simulink model "TSR_Scenario_001_cs"  (R2014b)
settings: Solver=ode5  SolverMode=SingleTasking  StartTime=0.0  StopTime=inf  FixedStep=1/100  RelTol=1e-3
PreLoadFcn:
  | mbxruntime.callbacks.PreLoadFcn(bdroot);
  | check_NUTS_defined;
  | 
  | assignin('base',['model_closed_' bdroot],false);
  | 
  | addpath('../includes_TSR/includes_TSR');
  | 
  | switch version('-release')
  | case {'2010a', '2010b', '2011a'}
  | addpath('../includes_TSR/ML2010b');
  | otherwise
  | addpath('../includes_TSR/ML2011b');
  | end
PostLoadFcn:
  | mbxruntime.callbacks.PostLoadFcn(bdroot);
InitFcn:
  | mbxruntime.callbacks.InitFcn(bdroot);
StartFcn:
  | mbxruntime.callbacks.StartFcn(bdroot);
StopFcn:
  | mbxruntime.callbacks.StopFcn(bdroot);
model workspace: external: MAT-File .\TSR_Scenario_001_cs_hws.mat (data not in the file)
undefined symbols (not defined in the file or in its folder): InitImageOutputDir, mbxruntime, OrientationPitch, OrientationRoll, PositionX, PositionY, PositionZ, tabledata, warningInitialVelocity, x0
undefined symbols (not defined in the file): SteeringColumn, SteeringWheel, TSR_Scenario_001_cs_0469e6db089af631, TSR_Scenario_001_cs_0511100212e7bc8e, TSR_Scenario_001_cs_0e7e9ae969427aac, TSR_Scenario_001_cs_1093386e49c2fe1f, TSR_Scenario_001_cs_112063adae8cf595, TSR_Scenario_001_cs_20f00d93cd5331c2, TSR_Scenario_001_cs_23e3512474fbfadc, TSR_Scenario_001_cs_366523e1554c6bf4, TSR_Scenario_001_cs_37bce4982c67337a, TSR_Scenario_001_cs_44e6164a5df50f45, TSR_Scenario_001_cs_4963ce12e7ff3247, TSR_Scenario_001_cs_4b3e01fa729ce73a, TSR_Scenario_001_cs_519c34727ce9f069, TSR_Scenario_001_cs_5b66ab60038399a1, TSR_Scenario_001_cs_5baa165dfa1afdcb, TSR_Scenario_001_cs_5f993ce39fa6372c, TSR_Scenario_001_cs_613fdf28e3ff7437, TSR_Scenario_001_cs_67b1406af835d622, TSR_Scenario_001_cs_6ad990c290286b94, TSR_Scenario_001_cs_6c412b69295984e1, TSR_Scenario_001_cs_6d4c0c06b1585ef3, TSR_Scenario_001_cs_6dd019d071bf1235, TSR_Scenario_001_cs_6e9f5883f1a78533, TSR_Scenario_001_cs_80f7223d9ac35404, TSR_Scenario_001_cs_8562b82d3c89ae57, TSR_Scenario_001_cs_8a3a0181ab0babfe, TSR_Scenario_001_cs_8c997348ce80deaf, TSR_Scenario_001_cs_925bd6a073d9fe25, TSR_Scenario_001_cs_961436216add6114, TSR_Scenario_001_cs_991a7959256b2c84, TSR_Scenario_001_cs_9a95ce2c2e753616, TSR_Scenario_001_cs_a98aa9562e8552a9, TSR_Scenario_001_cs_ab44ae81dbfb58cd, TSR_Scenario_001_cs_Actros_2541_2_Path_pathUniqueID, TSR_Scenario_001_cs_ae74836ade6bff5a, TSR_Scenario_001_cs_Audi_A8_1_Dynamics_Simple_initialPitch, TSR_Scenario_001_cs_Audi_A8_1_Dynamics_Simple_initialRoll, TSR_Scenario_001_cs_Audi_A8_1_Dynamics_Simple_initialX, TSR_Scenario_001_cs_Audi_A8_1_Dynamics_Simple_initialY, TSR_Scenario_001_cs_Audi_A8_1_Dynamics_Simple_initialYaw, TSR_Scenario_001_cs_Audi_A8_1_Dynamics_Simple_initialZ, TSR_Scenario_001_cs_Audi_A8_2_Path_pathUniqueID, TSR_Scenario_001_cs_Audi_A8_2_SpeedProfile_speedProfileUniqueID, TSR_Scenario_001_cs_b2eca4eb2fce349a, TSR_Scenario_001_cs_b7bac209c1f2549f, TSR_Scenario_001_cs_bf3dccb66d3255a4, TSR_Scenario_001_cs_bf4c1a5315e3f716, TSR_Scenario_001_cs_BMW_Z3_1_Path_pathUniqueID, TSR_Scenario_001_cs_BMW_Z3_1_SpeedProfile_speedProfileUniqueID, TSR_Scenario_001_cs_BMW_Z3_2_Path_pathUniqueID, TSR_Scenario_001_cs_BMW_Z3_2_SpeedProfile_speedProfileUniqueID, TSR_Scenario_001_cs_c4c8fc4bdece03a9, TSR_Scenario_001_cs_c964c86aa54ad92e, TSR_Scenario_001_cs_cb64d1ef85329755, TSR_Scenario_001_cs_Citroen_C3_1_Path_pathUniqueID, TSR_Scenario_001_cs_Citroen_C3_2_Path_pathUniqueID, TSR_Scenario_001_cs_Citroen_C3_3_Path_pathUniqueID, TSR_Scenario_001_cs_Citroen_C3_4_Path_pathUniqueID ... (+25)
libraries: simulink x21, PreScanSimulinkLibrary x17, simulink_extras x13
(part 4 of 30)

== system TSR_Scenario_001_cs/Citroen_C3_4 ==
  SELF_Citroen_C3_4 : Inport  Tag=inport/SelfPort  OutDataTypeStr=Bus: PRESCAN_SELFSENSORDATA  PortDimensions=1  SampleTime=1/100  BusOutputAsStruct=on
  ColorRegion_Exterior_color : Constant  Tag=VisuLightConst  Value=[255 240 245]
  Ground_{1..6} (6 alike) : Ground
  JointGroup_WheelDisplacement_V2R : Subsystem  Tag=mux/Wheels  mask(PreScan Velocity to Wheel Angle Block:){TimeStep=1/100, TireRadius=0.29}
      mask prompts: TimeStep "Auto Assigned: Time Step [s]"; TireRadius "Tire Radius [m]"
      settings: DeleteFcn=PreScanBlockDeleteFcn;
      mask Display: disp('Velocity\nto\nWheelAngle')
  Path : S-Function  Tag=Path  LoadFcn=load('PrescanMotionData.mat')  FunctionName=sfun_Path  Parameters=uniqueID, pathUniqueID, timestep  EnableBusSupport=off  mask(Path){uniqueID=2027, pathUniqueID=TSR_Scenario_001_cs_Citroen_C3_4_Path_pathUniqueID, timestep=1/100}
      mask prompts: uniqueID "Object Unique ID"; pathUniqueID "Path Unique ID"; timestep "MATLAB timestep:"
      mask help:
      | The path block outputs the position along a given trajectory.
      |
      | For more information, please click Help.
      mask Help: eval('openHelp(312)')
      mask Display: image(imread('Path.png'))
  SELF_Demux : Subsystem  Tag=demux/SelfPort  mask(PreScan Demux Block:){}
      mask help:
      | The SELF port shows (state) information of the actor itself. The outputs are position in the experiment's axis system and the GPS coordinates, and the object's absolute velocity and compass heading.
      |
      | For more information, please click Help.
      settings: DeleteFcn=PreScanBlockDeleteFcn;
      mask Help: eval('openHelp(462)')
      mask Display:
      | port_label('output',1,'x [m]')
      | port_label('output',2,'y [m]')
      | port_label('output',3,'z [m]','texmode','on')
      | port_label('output',4,'Rotx [deg]','texmode','on')
      | port_label('output',5,'Roty [deg]','texmode','on')
      | port_label('output',6,'Rotz [deg]','texmode','on')
      | port_label('output',7,'GPS lat [deg]','texmode','on')
      | port_label('output',8,'GPS long [deg]','texmode','on')
      | port_label('output',9,'GPS alt [m]','texmode','on')
      | port_label('output',10,'Velocity [m/s]')
      | port_label('output',11,'Heading [deg]')
      | port_label('output',12,'Yaw rate [deg/s]')
  STATE_Citroen_C3_4_rc : RateTransition  Tag=mux_rc/StatePort  OutPortSampleTimeOpt=Inherit
  SpeedProfile : S-Function  Tag=SpeedProfile  LoadFcn=load('PrescanMotionData.mat')  FunctionName=sfun_SpeedProfile  Parameters=speedProfileUniqueID, timestep  EnableBusSupport=off  mask(SpeedProfile){speedProfileUniqueID=TSR_Scenario_001_cs_def3abf47cdc3734, timestep=1/100}
      mask prompts: speedProfileUniqueID "Speed Profile Unique ID"; timestep "MATLAB timestep:"
      mask help:
      | The speed profile block outputs the travelled distance, velocities and acceleration along a given path.
      |
      | For more information, please click Help.
      mask Help: eval('openHelp(312)')
      mask Display: image(imread('SpeedProfile.png'))
  Terminator_{1..11} (11 alike) : Terminator
  VISUColorRegion_Exterior_Mux : Subsystem  Tag=mux/MuxColorRegion  LoadFcn=load PrescanColorData  mask(PreScan User Interface: VisuTextureColor){}
      mask help:
      | The VisuTextureColor block provides a way to adapt the color of a vehicle.
      |
      | For more information, please click Help.
      settings: DeleteFcn=PreScanBlockDeleteFcn;
      mask Help: eval('openHelp(230)')
  WheelDisplacement_Mux : Subsystem  Tag=mux/JointGroup  mask(JointGroup){}
      mask help:
      | The JointGroup allows to control several Joints in one go, as defined for this particular model.
      | For more information, look in the PreScan manual in the section "Model Preparation Tool" -> "Joint Groups"
      |
      | For more information on the Joints simulink interface, press Help.
      mask Help: eval('openHelp(254)')
  STATE_Citroen_C3_4_bus : Outport  Tag=outport/StatePort  OutDataTypeStr=Bus: PRESCAN_STATEACTUATORDATA  PortDimensions=1  SampleTime=1/100
  WheelL0_Citroen_C3_4 : Outport  Tag=outport/JointActuator  Port=2  OutDataTypeStr=Bus: PRESCAN_POSE_DATA  SampleTime=1/100
  WheelL1_Citroen_C3_4 : Outport  Tag=outport/JointActuator  Port=3  OutDataTypeStr=Bus: PRESCAN_POSE_DATA  SampleTime=1/100
  WheelR0_Citroen_C3_4 : Outport  Tag=outport/JointActuator  Port=4  OutDataTypeStr=Bus: PRESCAN_POSE_DATA  SampleTime=1/100
  WheelR1_Citroen_C3_4 : Outport  Tag=outport/JointActuator  Port=5  OutDataTypeStr=Bus: PRESCAN_POSE_DATA  SampleTime=1/100
  VISUColorRegion_Exterior_Citroen_C3_4 : Outport  Tag=outport/ColorRegion  Port=6  OutDataTypeStr=Bus: PRESCAN_COLOR_DATA  PortDimensions=1  SampleTime=1/100
  wires:
  SELF_Demux/10(velocity [m/s]) -> JointGroup_WheelDisplacement_V2R/1(Velocity [m/s])
  STATE_Citroen_C3_4_rc/1 -> STATE_Citroen_C3_4_bus/1
  SpeedProfile/1 -> Path/1
  Path/1 -> STATE_Citroen_C3_4_rc/1
  SELF_Citroen_C3_4/1 -> SELF_Demux/1(SELF)
  WheelDisplacement_Mux/1(WheelL0_Citroen_C3_4) -> WheelL0_Citroen_C3_4/1
  WheelDisplacement_Mux/2(WheelL1_Citroen_C3_4) -> WheelL1_Citroen_C3_4/1
  WheelDisplacement_Mux/3(WheelR0_Citroen_C3_4) -> WheelR0_Citroen_C3_4/1
  WheelDisplacement_Mux/4(WheelR1_Citroen_C3_4) -> WheelR1_Citroen_C3_4/1
  JointGroup_WheelDisplacement_V2R/1(Rotation [rad]) -> WheelDisplacement_Mux/3(Rotation [rad])
  VISUColorRegion_Exterior_Mux/1(ColorRegion) -> VISUColorRegion_Exterior_Citroen_C3_4/1
  ColorRegion_Exterior_color/1 -> VISUColorRegion_Exterior_Mux/1(RGB [-,-,-])
  SELF_Demux/1(x [m]) -> Terminator_1/1
  SELF_Demux/2(y [m]) -> Terminator_2/1
  SELF_Demux/3(z [m]) -> Terminator_3/1
  SELF_Demux/4(rotx [deg]) -> Terminator_4/1
  SELF_Demux/5(roty [deg]) -> Terminator_5/1
  SELF_Demux/6(rotz [deg]) -> Terminator_6/1
  SELF_Demux/7(GPS lat [deg]) -> Terminator_7/1
  SELF_Demux/8(GPS long [deg]) -> Terminator_8/1
  SELF_Demux/9(GPS alt [m]) -> Terminator_9/1
  SELF_Demux/11(heading [deg]) -> Terminator_10/1
  SELF_Demux/12(yaw rate [deg/s]) -> Terminator_11/1
  Ground_1/1 -> WheelDisplacement_Mux/1(Steering Angle Front [rad])
  Ground_2/1 -> WheelDisplacement_Mux/2(Steering Angle Rear [rad])
  Ground_3/1 -> WheelDisplacement_Mux/4(zDisp FL [m])
  Ground_4/1 -> WheelDisplacement_Mux/5(zDisp FR [m])
  Ground_5/1 -> WheelDisplacement_Mux/6(zDisp RL [m])
  Ground_6/1 -> WheelDisplacement_Mux/7(zDisp RR [m])

== system TSR_Scenario_001_cs/ContainerTrailer_DoubleAxle_1 ==
  SELF_ContainerTrailer_DoubleAxle_1 : Inport  Tag=inport/SelfPort  OutDataTypeStr=Bus: PRESCAN_SELFSENSORDATA  PortDimensions=1  SampleTime=1/100  BusOutputAsStruct=on
  ArticulatedActor : S-Function  FunctionName=sfun_ArticulatedActor  Parameters=tractorUniqueID, trailerUniqueID, timestep  EnableBusSupport=off  mask(ArticulatedActor){tractorUniqueID=1580, trailerUniqueID=1582, timestep=1/100}
      mask prompts: tractorUniqueID "Tractor Unique ID"; trailerUniqueID "Trailer Unique ID"; timestep "MATLAB timestep:"
      mask help:
      | The articulated actor block outputs the trailer position.
      |
      | For more information, please click Help.
      mask Help: eval('openHelp(1300)')
      mask Display: image(imread('TrailerKinematics.png'))
  SELF_Demux : Subsystem  Tag=demux/SelfPort  mask(PreScan Demux Block:){}
      mask help:
      | The SELF port shows (state) information of the actor itself. The outputs are position in the experiment's axis system and the GPS coordinates, and the object's absolute velocity and compass heading.
      |
      | For more information, please click Help.
      settings: DeleteFcn=PreScanBlockDeleteFcn;
      mask Help: eval('openHelp(462)')
      mask Display:
      | port_label('output',1,'x [m]')
      | port_label('output',2,'y [m]')
      | port_label('output',3,'z [m]','texmode','on')
      | port_label('output',4,'Rotx [deg]','texmode','on')
      | port_label('output',5,'Roty [deg]','texmode','on')
      | port_label('output',6,'Rotz [deg]','texmode','on')
      | port_label('output',7,'GPS lat [deg]','texmode','on')
      | port_label('output',8,'GPS long [deg]','texmode','on')
      | port_label('output',9,'GPS alt [m]','texmode','on')
      | port_label('output',10,'Velocity [m/s]')
      | port_label('output',11,'Heading [deg]')
      | port_label('output',12,'Yaw rate [deg/s]')
  STATE_ContainerTrailer_DoubleAxle_1_rc : RateTransition  Tag=mux_rc/StatePort  OutPortSampleTimeOpt=Inherit
  Terminator_{1..12} (12 alike) : Terminator
  STATE_ContainerTrailer_DoubleAxle_1_bus : Outport  Tag=outport/StatePort  OutDataTypeStr=Bus: PRESCAN_STATEACTUATORDATA  PortDimensions=1  SampleTime=1/100
  wires:
  STATE_ContainerTrailer_DoubleAxle_1_rc/1 -> STATE_ContainerTrailer_DoubleAxle_1_bus/1
  SELF_ContainerTrailer_DoubleAxle_1/1 -> SELF_Demux/1(SELF)
  ArticulatedActor/1 -> STATE_ContainerTrailer_DoubleAxle_1_rc/1
  [Actros_1860_1_state] -> ArticulatedActor/1
  SELF_Demux/1(x [m]) -> Terminator_1/1
  SELF_Demux/2(y [m]) -> Terminator_2/1
  SELF_Demux/3(z [m]) -> Terminator_3/1
  SELF_Demux/4(rotx [deg]) -> Terminator_4/1
  SELF_Demux/5(roty [deg]) -> Terminator_5/1
  SELF_Demux/6(rotz [deg]) -> Terminator_6/1
  SELF_Demux/7(GPS lat [deg]) -> Terminator_7/1
  SELF_Demux/8(GPS long [deg]) -> Terminator_8/1
  SELF_Demux/9(GPS alt [m]) -> Terminator_9/1
  SELF_Demux/10(velocity [m/s]) -> Terminator_10/1
  SELF_Demux/11(heading [deg]) -> Terminator_11/1
  SELF_Demux/12(yaw rate [deg/s]) -> Terminator_12/1

== system TSR_Scenario_001_cs/ContainerTrailer_DoubleAxle_2 ==
  SELF_ContainerTrailer_DoubleAxle_2 : Inport  Tag=inport/SelfPort  OutDataTypeStr=Bus: PRESCAN_SELFSENSORDATA  PortDimensions=1  SampleTime=1/100  BusOutputAsStruct=on
  ArticulatedActor : S-Function  FunctionName=sfun_ArticulatedActor  Parameters=tractorUniqueID, trailerUniqueID, timestep  EnableBusSupport=off  mask(ArticulatedActor){tractorUniqueID=1584, trailerUniqueID=1586, timestep=1/100}
      mask prompts: tractorUniqueID "Tractor Unique ID"; trailerUniqueID "Trailer Unique ID"; timestep "MATLAB timestep:"
      mask help:
      | The articulated actor block outputs the trailer position.
      |
      | For more information, please click Help.
      mask Help: eval('openHelp(1300)')
      mask Display: image(imread('TrailerKinematics.png'))
  SELF_Demux : Subsystem  Tag=demux/SelfPort  mask(PreScan Demux Block:){}
      mask help:
      | The SELF port shows (state) information of the actor itself. The outputs are position in the experiment's axis system and the GPS coordinates, and the object's absolute velocity and compass heading.
      |
      | For more information, please click Help.
      settings: DeleteFcn=PreScanBlockDeleteFcn;
      mask Help: eval('openHelp(462)')
      mask Display:
      | port_label('output',1,'x [m]')
      | port_label('output',2,'y [m]')
      | port_label('output',3,'z [m]','texmode','on')
      | port_label('output',4,'Rotx [deg]','texmode','on')
      | port_label('output',5,'Roty [deg]','texmode','on')
      | port_label('output',6,'Rotz [deg]','texmode','on')
      | port_label('output',7,'GPS lat [deg]','texmode','on')
      | port_label('output',8,'GPS long [deg]','texmode','on')
      | port_label('output',9,'GPS alt [m]','texmode','on')
      | port_label('output',10,'Velocity [m/s]')
      | port_label('output',11,'Heading [deg]')
      | port_label('output',12,'Yaw rate [deg/s]')
  STATE_ContainerTrailer_DoubleAxle_2_rc : RateTransition  Tag=mux_rc/StatePort  OutPortSampleTimeOpt=Inherit
  Terminator_{1..12} (12 alike) : Terminator
  STATE_ContainerTrailer_DoubleAxle_2_bus : Outport  Tag=outport/StatePort  OutDataTypeStr=Bus: PRESCAN_STATEACTUATORDATA  PortDimensions=1  SampleTime=1/100
  wires:
  STATE_ContainerTrailer_DoubleAxle_2_rc/1 -> STATE_ContainerTrailer_DoubleAxle_2_bus/1
  SELF_ContainerTrailer_DoubleAxle_2/1 -> SELF_Demux/1(SELF)
  ArticulatedActor/1 -> STATE_ContainerTrailer_DoubleAxle_2_rc/1
  [Actros_1860_2_state] -> ArticulatedActor/1
  SELF_Demux/1(x [m]) -> Terminator_1/1
  SELF_Demux/2(y [m]) -> Terminator_2/1
  SELF_Demux/3(z [m]) -> Terminator_3/1
  SELF_Demux/4(rotx [deg]) -> Terminator_4/1
  SELF_Demux/5(roty [deg]) -> Terminator_5/1
  SELF_Demux/6(rotz [deg]) -> Terminator_6/1
  SELF_Demux/7(GPS lat [deg]) -> Terminator_7/1
  SELF_Demux/8(GPS long [deg]) -> Terminator_8/1
  SELF_Demux/9(GPS alt [m]) -> Terminator_9/1
  SELF_Demux/10(velocity [m/s]) -> Terminator_10/1
  SELF_Demux/11(heading [deg]) -> Terminator_11/1
  SELF_Demux/12(yaw rate [deg/s]) -> Terminator_12/1

== system TSR_Scenario_001_cs/Controller ==
  Terminator : Terminator
  sfun_Controller : S-Function  FunctionName=sfun_Controller  Parameters=SParameter1, SParameter2, SParameter3, SParameter4, SParameter5, SParameter6, SParameter7, SParameter8, SParameter9, SParameter10, SampleTime  EnableBusSupport=off  mask(Legacy Function){SFunctionSpec=void prescan_outputFcn(void** work1, PRESCAN_CONTROLLERDATA y1[1]), SParameter1=uint8([ExperimentFile 0]), SParameter2=uint8([ModelDepo 0]), SParameter3=uint8([ControllerOptions 0]), SParameter4=RTmode, SParameter5=PreScanExecutionMode, SParameter6=ControlMode, SParameter7=ControllerCount, SParameter8=ControllerIndex, SParameter9=uint8([SimulationMode 0]), SParameter10=uint8([TargetName 0]), SampleTime=TimeStep, ShowSpec=on}
      mask prompts: SParameter1 "P1:"; SParameter2 "P2:"; SParameter3 "P3:"; SParameter4 "P4:"; SParameter5 "P5:"; SParameter6 "P6:"; SParameter7 "P7:"; SParameter8 "P8:"; SParameter9 "P9:"; SParameter10 "P10:"; SampleTime "Sample time (-1 for inherited):"; ShowSpec "Display function specification"
      mask help:
      | This block allows you to call the legacy functions specified by the following Legacy Code Tool definition:
      | def.SFunctionName = 'sfun_Controller';
      | def.OutputFcnSpec = 'void prescan_outputFcn(void** work1, PRESCAN_CONTROLLERDATA y1[1])';
      | def.StartFcnSpec = 'void prescan_startFcn(void ** work1, uint8 p1[], uint8 p2[], uint8 p3[], double p4, double p5, double p6, double p7, double p8, uint8 p9[], uint8 p10[])';
      | def.TerminateFcnSpec = 'void prescan_terminateFcn(void** work1)';
      | def.HeaderFiles = {'prescan_controller_data.h', 'prescan_SFunLibrary.h', 'prescan_CreateLogHandler.h', 'prescan_CreateErrorHandler.h', 'prescan_modify.h', 'ModuleDLL.h'};
      | def.SourceFiles = {'prescan_MexLogHandler.c', 'prescan_SimStructErrorHandler.c', 'prescan_LogHandler.c', 'prescan_ErrorHandler.c', 'prescan_Modify.c'};
      | def.HostLibFiles = {'sensorinterfaced.lib'};
      | def.TargetLibFiles = {'sensorinterfaced.so'};
      | def.IncPaths = {'.', 'C:\projects\prescan\rt_vislibrary\vis\..\pimp\include\sensors\InterfaceRTW'};
      | def.SrcPaths = {'C:\projects\prescan\rt_vislibrary\vis\..\pimp\include\sensors\InterfaceRTW', 'C:\projects\prescan\rt_vislibrary\vis\..\pimp\include\sensors\InterfaceRTW\ccurrt'};
      | def.LibPaths = {'C:\\projects\\prescan\\vislibrary_build\lib'};
      | def.SampleTime = 'parameterized';
      mask Help: <p>This block was generated automatically by the Legacy Code Tool. For detailed help on this tool, call<a href="matlab:legacy_code('help')"> legacy_code('help')</a>.</p>
      mask Callback ShowSpec:
      | if strcmp(get_param(gcbh, 'ShowSpec'), 'on')
      |   set_param(gcbh, 'MaskDisplay', sprintf('fprintf(''%s'');', get_param(gcbh, 'SFunctionSpec')));
      | else
      |   set_param(gcbh, 'MaskDisplay', sprintf('fprintf(''%s'');', get_param(gcbh, 'FunctionName')));
      | end
      mask Display: fprintf('void prescan_outputFcn(void** work1, PRESCAN_CONTROLLERDATA y1[1])');
  wires:
  sfun_Controller/1 -> Terminator/1

== system TSR_Scenario_001_cs/Fiat_Bravo_1 ==
  SELF_Fiat_Bravo_1 : Inport  Tag=inport/SelfPort  OutDataTypeStr=Bus: PRESCAN_SELFSENSORDATA  PortDimensions=1  SampleTime=1/100  BusOutputAsStruct=on
  ColorRegion_Exterior_color : Constant  Tag=VisuLightConst  Value=[0 191 255]
  Ground_{1..6} (6 alike) : Ground
  JointGroup_WheelDisplacement_V2R : Subsystem  Tag=mux/Wheels  mask(PreScan Velocity to Wheel Angle Block:){TimeStep=1/100, TireRadius=0.29}
      mask prompts: TimeStep "Auto Assigned: Time Step [s]"; TireRadius "Tire Radius [m]"
      settings: DeleteFcn=PreScanBlockDeleteFcn;
      mask Display: disp('Velocity\nto\nWheelAngle')
  Path : S-Function  Tag=Path  LoadFcn=load('PrescanMotionData.mat')  FunctionName=sfun_Path  Parameters=uniqueID, pathUniqueID, timestep  EnableBusSupport=off  mask(Path){uniqueID=1964, pathUniqueID=TSR_Scenario_001_cs_Fiat_Bravo_1_Path_pathUniqueID, timestep=1/100}
      mask prompts: uniqueID "Object Unique ID"; pathUniqueID "Path Unique ID"; timestep "MATLAB timestep:"
      mask help:
      | The path block outputs the position along a given trajectory.
      |
      | For more information, please click Help.
      mask Help: eval('openHelp(312)')
      mask Display: image(imread('Path.png'))
  SELF_Demux : Subsystem  Tag=demux/SelfPort  mask(PreScan Demux Block:){}
      mask help:
      | The SELF port shows (state) information of the actor itself. The outputs are position in the experiment's axis system and the GPS coordinates, and the object's absolute velocity and compass heading.
      |
      | For more information, please click Help.
      settings: DeleteFcn=PreScanBlockDeleteFcn;
      mask Help: eval('openHelp(462)')
      mask Display:
      | port_label('output',1,'x [m]')
      | port_label('output',2,'y [m]')
      | port_label('output',3,'z [m]','texmode','on')
      | port_label('output',4,'Rotx [deg]','texmode','on')
      | port_label('output',5,'Roty [deg]','texmode','on')
      | port_label('output',6,'Rotz [deg]','texmode','on')
      | port_label('output',7,'GPS lat [deg]','texmode','on')
      | port_label('output',8,'GPS long [deg]','texmode','on')
      | port_label('output',9,'GPS alt [m]','texmode','on')
      | port_label('output',10,'Velocity [m/s]')
      | port_label('output',11,'Heading [deg]')
      | port_label('output',12,'Yaw rate [deg/s]')
  STATE_Fiat_Bravo_1_rc : RateTransition  Tag=mux_rc/StatePort  OutPortSampleTimeOpt=Inherit
  SpeedProfile : S-Function  Tag=SpeedProfile  LoadFcn=load('PrescanMotionData.mat')  FunctionName=sfun_SpeedProfile  Parameters=speedProfileUniqueID, timestep  EnableBusSupport=off  mask(SpeedProfile){speedProfileUniqueID=TSR_Scenario_001_cs_fb6cb42c10e88917, timestep=1/100}
      mask prompts: speedProfileUniqueID "Speed Profile Unique ID"; timestep "MATLAB timestep:"
      mask help:
      | The speed profile block outputs the travelled distance, velocities and acceleration along a given path.
      |
      | For more information, please click Help.
      mask Help: eval('openHelp(312)')
      mask Display: image(imread('SpeedProfile.png'))
  Terminator_{1..11} (11 alike) : Terminator
  VISUColorRegion_Exterior_Mux : Subsystem  Tag=mux/MuxColorRegion  LoadFcn=load PrescanColorData  mask(PreScan User Interface: VisuTextureColor){}
      mask help:
      | The VisuTextureColor block provides a way to adapt the color of a vehicle.
      |
      | For more information, please click Help.
      settings: DeleteFcn=PreScanBlockDeleteFcn;
      mask Help: eval('openHelp(230)')
  WheelDisplacement_Mux : Subsystem  Tag=mux/JointGroup  mask(JointGroup){}
      mask help:
      | The JointGroup allows to control several Joints in one go, as defined for this particular model.
      | For more information, look in the PreScan manual in the section "Model Preparation Tool" -> "Joint Groups"
      |
      | For more information on the Joints simulink interface, press Help.
      mask Help: eval('openHelp(254)')
  STATE_Fiat_Bravo_1_bus : Outport  Tag=outport/StatePort  OutDataTypeStr=Bus: PRESCAN_STATEACTUATORDATA  PortDimensions=1  SampleTime=1/100
  WheelL0_Fiat_Bravo_1 : Outport  Tag=outport/JointActuator  Port=2  OutDataTypeStr=Bus: PRESCAN_POSE_DATA  SampleTime=1/100
  WheelL1_Fiat_Bravo_1 : Outport  Tag=outport/JointActuator  Port=3  OutDataTypeStr=Bus: PRESCAN_POSE_DATA  SampleTime=1/100
  WheelR0_Fiat_Bravo_1 : Outport  Tag=outport/JointActuator  Port=4  OutDataTypeStr=Bus: PRESCAN_POSE_DATA  SampleTime=1/100
  WheelR1_Fiat_Bravo_1 : Outport  Tag=outport/JointActuator  Port=5  OutDataTypeStr=Bus: PRESCAN_POSE_DATA  SampleTime=1/100
  VISUColorRegion_Exterior_Fiat_Bravo_1 : Outport  Tag=outport/ColorRegion  Port=6  OutDataTypeStr=Bus: PRESCAN_COLOR_DATA  PortDimensions=1  SampleTime=1/100
  wires:
  SELF_Demux/10(velocity [m/s]) -> JointGroup_WheelDisplacement_V2R/1(Velocity [m/s])
  STATE_Fiat_Bravo_1_rc/1 -> STATE_Fiat_Bravo_1_bus/1
  SpeedProfile/1 -> Path/1
  Path/1 -> STATE_Fiat_Bravo_1_rc/1
  SELF_Fiat_Bravo_1/1 -> SELF_Demux/1(SELF)
  WheelDisplacement_Mux/1(WheelL0_Fiat_Bravo_1) -> WheelL0_Fiat_Bravo_1/1
  WheelDisplacement_Mux/2(WheelL1_Fiat_Bravo_1) -> WheelL1_Fiat_Bravo_1/1
  WheelDisplacement_Mux/3(WheelR0_Fiat_Bravo_1) -> WheelR0_Fiat_Bravo_1/1
  WheelDisplacement_Mux/4(WheelR1_Fiat_Bravo_1) -> WheelR1_Fiat_Bravo_1/1
  JointGroup_WheelDisplacement_V2R/1(Rotation [rad]) -> WheelDisplacement_Mux/3(Rotation [rad])
  VISUColorRegion_Exterior_Mux/1(ColorRegion) -> VISUColorRegion_Exterior_Fiat_Bravo_1/1
  ColorRegion_Exterior_color/1 -> VISUColorRegion_Exterior_Mux/1(RGB [-,-,-])
  SELF_Demux/1(x [m]) -> Terminator_1/1
  SELF_Demux/2(y [m]) -> Terminator_2/1
  SELF_Demux/3(z [m]) -> Terminator_3/1
  SELF_Demux/4(rotx [deg]) -> Terminator_4/1
  SELF_Demux/5(roty [deg]) -> Terminator_5/1
  SELF_Demux/6(rotz [deg]) -> Terminator_6/1
  SELF_Demux/7(GPS lat [deg]) -> Terminator_7/1
  SELF_Demux/8(GPS long [deg]) -> Terminator_8/1
  SELF_Demux/9(GPS alt [m]) -> Terminator_9/1
  SELF_Demux/11(heading [deg]) -> Terminator_10/1
  SELF_Demux/12(yaw rate [deg/s]) -> Terminator_11/1
  Ground_1/1 -> WheelDisplacement_Mux/1(Steering Angle Front [rad])
  Ground_2/1 -> WheelDisplacement_Mux/2(Steering Angle Rear [rad])
  Ground_3/1 -> WheelDisplacement_Mux/4(zDisp FL [m])
  Ground_4/1 -> WheelDisplacement_Mux/5(zDisp FR [m])
  Ground_5/1 -> WheelDisplacement_Mux/6(zDisp RL [m])
  Ground_6/1 -> WheelDisplacement_Mux/7(zDisp RR [m])

== system TSR_Scenario_001_cs/Fiat_Bravo_2 ==
  SELF_Fiat_Bravo_2 : Inport  Tag=inport/SelfPort  OutDataTypeStr=Bus: PRESCAN_SELFSENSORDATA  PortDimensions=1  SampleTime=1/100  BusOutputAsStruct=on
  Ground_{1..6} (6 alike) : Ground
  JointGroup_WheelDisplacement_V2R : Subsystem  Tag=mux/Wheels  mask(PreScan Velocity to Wheel Angle Block:){TimeStep=1/100, TireRadius=0.29}
      mask prompts: TimeStep "Auto Assigned: Time Step [s]"; TireRadius "Tire Radius [m]"
      settings: DeleteFcn=PreScanBlockDeleteFcn;
      mask Display: disp('Velocity\nto\nWheelAngle')
  Path : S-Function  Tag=Path  LoadFcn=load('PrescanMotionData.mat')  FunctionName=sfun_Path  Parameters=uniqueID, pathUniqueID, timestep  EnableBusSupport=off  mask(Path){uniqueID=2021, pathUniqueID=TSR_Scenario_001_cs_Fiat_Bravo_2_Path_pathUniqueID, timestep=1/100}
      mask prompts: uniqueID "Object Unique ID"; pathUniqueID "Path Unique ID"; timestep "MATLAB timestep:"
      mask help:
      | The path block outputs the position along a given trajectory.
      |
      | For more information, please click Help.
      mask Help: eval('openHelp(312)')
      mask Display: image(imread('Path.png'))
  SELF_Demux : Subsystem  Tag=demux/SelfPort  mask(PreScan Demux Block:){}
      mask help:
      | The SELF port shows (state) information of the actor itself. The outputs are position in the experiment's axis system and the GPS coordinates, and the object's absolute velocity and compass heading.
      |
      | For more information, please click Help.
      settings: DeleteFcn=PreScanBlockDeleteFcn;
      mask Help: eval('openHelp(462)')
      mask Display:
      | port_label('output',1,'x [m]')
      | port_label('output',2,'y [m]')
      | port_label('output',3,'z [m]','texmode','on')
      | port_label('output',4,'Rotx [deg]','texmode','on')
      | port_label('output',5,'Roty [deg]','texmode','on')
      | port_label('output',6,'Rotz [deg]','texmode','on')
      | port_label('output',7,'GPS lat [deg]','texmode','on')
      | port_label('output',8,'GPS long [deg]','texmode','on')
      | port_label('output',9,'GPS alt [m]','texmode','on')
      | port_label('output',10,'Velocity [m/s]')
      | port_label('output',11,'Heading [deg]')
      | port_label('output',12,'Yaw rate [deg/s]')
  STATE_Fiat_Bravo_2_rc : RateTransition  Tag=mux_rc/StatePort  OutPortSampleTimeOpt=Inherit
  SpeedProfile : S-Function  Tag=SpeedProfile  LoadFcn=load('PrescanMotionData.mat')  FunctionName=sfun_SpeedProfile  Parameters=speedProfileUniqueID, timestep  EnableBusSupport=off  mask(SpeedProfile){speedProfileUniqueID=TSR_Scenario_001_cs_fd67c8a405d181e0, timestep=1/100}
      mask prompts: speedProfileUniqueID "Speed Profile Unique ID"; timestep "MATLAB timestep:"
      mask help:
      | The speed profile block outputs the travelled distance, velocities and acceleration along a given path.
      |
      | For more information, please click Help.
      mask Help: eval('openHelp(312)')
      mask Display: image(imread('SpeedProfile.png'))
  Terminator_{1..11} (11 alike) : Terminator
  WheelDisplacement_Mux : Subsystem  Tag=mux/JointGroup  mask(JointGroup){}
      mask help:
      | The JointGroup allows to control several Joints in one go, as defined for this particular model.
      | For more information, look in the PreScan manual in the section "Model Preparation Tool" -> "Joint Groups"
      |
      | For more information on the Joints simulink interface, press Help.
      mask Help: eval('openHelp(254)')
  STATE_Fiat_Bravo_2_bus : Outport  Tag=outport/StatePort  OutDataTypeStr=Bus: PRESCAN_STATEACTUATORDATA  PortDimensions=1  SampleTime=1/100
  WheelL0_Fiat_Bravo_2 : Outport  Tag=outport/JointActuator  Port=2  OutDataTypeStr=Bus: PRESCAN_POSE_DATA  SampleTime=1/100
  WheelL1_Fiat_Bravo_2 : Outport  Tag=outport/JointActuator  Port=3  OutDataTypeStr=Bus: PRESCAN_POSE_DATA  SampleTime=1/100
  WheelR0_Fiat_Bravo_2 : Outport  Tag=outport/JointActuator  Port=4  OutDataTypeStr=Bus: PRESCAN_POSE_DATA  SampleTime=1/100
  WheelR1_Fiat_Bravo_2 : Outport  Tag=outport/JointActuator  Port=5  OutDataTypeStr=Bus: PRESCAN_POSE_DATA  SampleTime=1/100
  wires:
  SELF_Demux/10(velocity [m/s]) -> JointGroup_WheelDisplacement_V2R/1(Velocity [m/s])
  STATE_Fiat_Bravo_2_rc/1 -> STATE_Fiat_Bravo_2_bus/1
  SpeedProfile/1 -> Path/1
  Path/1 -> STATE_Fiat_Bravo_2_rc/1
  SELF_Fiat_Bravo_2/1 -> SELF_Demux/1(SELF)
  WheelDisplacement_Mux/1(WheelL0_Fiat_Bravo_2) -> WheelL0_Fiat_Bravo_2/1
  WheelDisplacement_Mux/2(WheelL1_Fiat_Bravo_2) -> WheelL1_Fiat_Bravo_2/1
  WheelDisplacement_Mux/3(WheelR0_Fiat_Bravo_2) -> WheelR0_Fiat_Bravo_2/1
  WheelDisplacement_Mux/4(WheelR1_Fiat_Bravo_2) -> WheelR1_Fiat_Bravo_2/1
  JointGroup_WheelDisplacement_V2R/1(Rotation [rad]) -> WheelDisplacement_Mux/3(Rotation [rad])
  SELF_Demux/1(x [m]) -> Terminator_1/1
  SELF_Demux/2(y [m]) -> Terminator_2/1
  SELF_Demux/3(z [m]) -> Terminator_3/1
  SELF_Demux/4(rotx [deg]) -> Terminator_4/1
  SELF_Demux/5(roty [deg]) -> Terminator_5/1
  SELF_Demux/6(rotz [deg]) -> Terminator_6/1
  SELF_Demux/7(GPS lat [deg]) -> Terminator_7/1
  SELF_Demux/8(GPS long [deg]) -> Terminator_8/1
  SELF_Demux/9(GPS alt [m]) -> Terminator_9/1
  SELF_Demux/11(heading [deg]) -> Terminator_10/1
  SELF_Demux/12(yaw rate [deg/s]) -> Terminator_11/1
  Ground_1/1 -> WheelDisplacement_Mux/1(Steering Angle Front [rad])
  Ground_2/1 -> WheelDisplacement_Mux/2(Steering Angle Rear [rad])
  Ground_3/1 -> WheelDisplacement_Mux/4(zDisp FL [m])
  Ground_4/1 -> WheelDisplacement_Mux/5(zDisp FR [m])
  Ground_5/1 -> WheelDisplacement_Mux/6(zDisp RL [m])
  Ground_6/1 -> WheelDisplacement_Mux/7(zDisp RR [m])

== system TSR_Scenario_001_cs/Ford_Fiesta_1 ==
  SELF_Ford_Fiesta_1 : Inport  Tag=inport/SelfPort  OutDataTypeStr=Bus: PRESCAN_SELFSENSORDATA  PortDimensions=1  SampleTime=1/100  BusOutputAsStruct=on
  ColorRegion_Exterior_color : Constant  Tag=VisuLightConst  Value=[210 105 30]
  Ground_{1..6} (6 alike) : Ground
  JointGroup_WheelDisplacement_V2R : Subsystem  Tag=mux/Wheels  mask(PreScan Velocity to Wheel Angle Block:){TimeStep=1/100, TireRadius=0.29}
      mask prompts: TimeStep "Auto Assigned: Time Step [s]"; TireRadius "Tire Radius [m]"
      settings: DeleteFcn=PreScanBlockDeleteFcn;
      mask Display: disp('Velocity\nto\nWheelAngle')
  Path : S-Function  Tag=Path  LoadFcn=load('PrescanMotionData.mat')  FunctionName=sfun_Path  Parameters=uniqueID, pathUniqueID, timestep  EnableBusSupport=off  mask(Path){uniqueID=1934, pathUniqueID=TSR_Scenario_001_cs_Ford_Fiesta_1_Path_pathUniqueID, timestep=1/100}
      mask prompts: uniqueID "Object Unique ID"; pathUniqueID "Path Unique ID"; timestep "MATLAB timestep:"
      mask help:
      | The path block outputs the position along a given trajectory.
      |
      | For more information, please click Help.
      mask Help: eval('openHelp(312)')
      mask Display: image(imread('Path.png'))
  SELF_Demux : Subsystem  Tag=demux/SelfPort  mask(PreScan Demux Block:){}
      mask help:
      | The SELF port shows (state) information of the actor itself. The outputs are position in the experiment's axis system and the GPS coordinates, and the object's absolute velocity and compass heading.
      |
      | For more information, please click Help.
      settings: DeleteFcn=PreScanBlockDeleteFcn;
      mask Help: eval('openHelp(462)')
      mask Display:
      | port_label('output',1,'x [m]')
      | port_label('output',2,'y [m]')
      | port_label('output',3,'z [m]','texmode','on')
      | port_label('output',4,'Rotx [deg]','texmode','on')
      | port_label('output',5,'Roty [deg]','texmode','on')
      | port_label('output',6,'Rotz [deg]','texmode','on')
      | port_label('output',7,'GPS lat [deg]','texmode','on')
      | port_label('output',8,'GPS long [deg]','texmode','on')
      | port_label('output',9,'GPS alt [m]','texmode','on')
      | port_label('output',10,'Velocity [m/s]')
      | port_label('output',11,'Heading [deg]')
      | port_label('output',12,'Yaw rate [deg/s]')
  STATE_Ford_Fiesta_1_rc : RateTransition  Tag=mux_rc/StatePort  OutPortSampleTimeOpt=Inherit
  SpeedProfile : S-Function  Tag=SpeedProfile  LoadFcn=load('PrescanMotionData.mat')  FunctionName=sfun_SpeedProfile  Parameters=speedProfileUniqueID, timestep  EnableBusSupport=off  mask(SpeedProfile){speedProfileUniqueID=TSR_Scenario_001_cs_c964c86aa54ad92e, timestep=1/100}
      mask prompts: speedProfileUniqueID "Speed Profile Unique ID"; timestep "MATLAB timestep:"
      mask help:
      | The speed profile block outputs the travelled distance, velocities and acceleration along a given path.
      |
      | For more information, please click Help.
      mask Help: eval('openHelp(312)')
      mask Display: image(imread('SpeedProfile.png'))
  Terminator_{1..11} (11 alike) : Terminator
  VISUColorRegion_Exterior_Mux : Subsystem  Tag=mux/MuxColorRegion  LoadFcn=load PrescanColorData  mask(PreScan User Interface: VisuTextureColor){}
      mask help:
      | The VisuTextureColor block provides a way to adapt the color of a vehicle.
      |
      | For more information, please click Help.
      settings: DeleteFcn=PreScanBlockDeleteFcn;
      mask Help: eval('openHelp(230)')
  WheelDisplacement_Mux : Subsystem  Tag=mux/JointGroup  mask(JointGroup){}
      mask help:
      | The JointGroup allows to control several Joints in one go, as defined for this particular model.
      | For more information, look in the PreScan manual in the section "Model Preparation Tool" -> "Joint Groups"
      |
      | For more information on the Joints simulink interface, press Help.
      mask Help: eval('openHelp(254)')
  STATE_Ford_Fiesta_1_bus : Outport  Tag=outport/StatePort  OutDataTypeStr=Bus: PRESCAN_STATEACTUATORDATA  PortDimensions=1  SampleTime=1/100
  WheelL0_Ford_Fiesta_1 : Outport  Tag=outport/JointActuator  Port=2  OutDataTypeStr=Bus: PRESCAN_POSE_DATA  SampleTime=1/100
  WheelL1_Ford_Fiesta_1 : Outport  Tag=outport/JointActuator  Port=3  OutDataTypeStr=Bus: PRESCAN_POSE_DATA  SampleTime=1/100
  WheelR0_Ford_Fiesta_1 : Outport  Tag=outport/JointActuator  Port=4  OutDataTypeStr=Bus: PRESCAN_POSE_DATA  SampleTime=1/100
  WheelR1_Ford_Fiesta_1 : Outport  Tag=outport/JointActuator  Port=5  OutDataTypeStr=Bus: PRESCAN_POSE_DATA  SampleTime=1/100
  VISUColorRegion_Exterior_Ford_Fiesta_1 : Outport  Tag=outport/ColorRegion  Port=6  OutDataTypeStr=Bus: PRESCAN_COLOR_DATA  PortDimensions=1  SampleTime=1/100
  wires:
  SELF_Demux/10(velocity [m/s]) -> JointGroup_WheelDisplacement_V2R/1(Velocity [m/s])
  STATE_Ford_Fiesta_1_rc/1 -> STATE_Ford_Fiesta_1_bus/1
  SpeedProfile/1 -> Path/1
  Path/1 -> STATE_Ford_Fiesta_1_rc/1
  SELF_Ford_Fiesta_1/1 -> SELF_Demux/1(SELF)
  WheelDisplacement_Mux/1(WheelL0_Ford_Fiesta_1) -> WheelL0_Ford_Fiesta_1/1
  WheelDisplacement_Mux/2(WheelL1_Ford_Fiesta_1) -> WheelL1_Ford_Fiesta_1/1
  WheelDisplacement_Mux/3(WheelR0_Ford_Fiesta_1) -> WheelR0_Ford_Fiesta_1/1
  WheelDisplacement_Mux/4(WheelR1_Ford_Fiesta_1) -> WheelR1_Ford_Fiesta_1/1
  JointGroup_WheelDisplacement_V2R/1(Rotation [rad]) -> WheelDisplacement_Mux/3(Rotation [rad])
  VISUColorRegion_Exterior_Mux/1(ColorRegion) -> VISUColorRegion_Exterior_Ford_Fiesta_1/1
  ColorRegion_Exterior_color/1 -> VISUColorRegion_Exterior_Mux/1(RGB [-,-,-])
  SELF_Demux/1(x [m]) -> Terminator_1/1
  SELF_Demux/2(y [m]) -> Terminator_2/1
  SELF_Demux/3(z [m]) -> Terminator_3/1
  SELF_Demux/4(rotx [deg]) -> Terminator_4/1
  SELF_Demux/5(roty [deg]) -> Terminator_5/1
  SELF_Demux/6(rotz [deg]) -> Terminator_6/1
  SELF_Demux/7(GPS lat [deg]) -> Terminator_7/1
  SELF_Demux/8(GPS long [deg]) -> Terminator_8/1
  SELF_Demux/9(GPS alt [m]) -> Terminator_9/1
  SELF_Demux/11(heading [deg]) -> Terminator_10/1
  SELF_Demux/12(yaw rate [deg/s]) -> Terminator_11/1
  Ground_1/1 -> WheelDisplacement_Mux/1(Steering Angle Front [rad])
  Ground_2/1 -> WheelDisplacement_Mux/2(Steering Angle Rear [rad])
  Ground_3/1 -> WheelDisplacement_Mux/4(zDisp FL [m])
  Ground_4/1 -> WheelDisplacement_Mux/5(zDisp FR [m])
  Ground_5/1 -> WheelDisplacement_Mux/6(zDisp RL [m])
  Ground_6/1 -> WheelDisplacement_Mux/7(zDisp RR [m])

== system TSR_Scenario_001_cs/HighwayOverhang_1 ==
  note: Resources
      |
      | 3: InformationSign\MatrixSign_Empty.png: MatrixSign Empty
      | 4: InformationSign\MatrixSign_End.png: MatrixSign End
      | 5: InformationSign\MatrixSign_GreenArrow.png: MatrixSign GreenArrow
      | 6: InformationSign\MatrixSign_RedCross.png: MatrixSign RedCross
      | 7: InformationSign\MatrixSign_Speed_50.png: MatrixSign Speed 50
      | 8: InformationSign\MatrixSign_Speed_70.png: MatrixSign Speed 70
      | 9: InformationSign\MatrixSign_Speed_90.png: MatrixSign Speed 90
      | 10: InformationSign\MatrixSign_Speed_120.png: MatrixSign Speed 120
      | 11: InformationSign\MatrixSign_Speed_130.png: MatrixSign Speed 130
      | 12: InformationSign\information.png: information
      | 13: InformationSign\Empty.jpg: Empty
  Ground_{1..8} (8 alike) : Ground
  VISUMatrixSignLights_Mux : Subsystem  Tag=mux/VisuMatrixSignLights  mask(PreScan User Interface: VisuMatrixSignLights){}
      mask help:
      | The VisuMatrixSignLights block provides a way to switch the lights on the matrix sign board on or off
      |
      | For more information, please click Help.
      mask Help: eval('openHelp(732)')
  VISUMatrixSign_Mux : Subsystem  Tag=mux/MatrixSign_v2  mask(PreScan User Interface: VisuMatrixSign){}
      mask help:
      | The VisuMatrixSign block provides a way to adapt the texture of the plates connected to an overhang, based on Resource IDs of the texture files.
      |
      | For more information, please click Help.
      settings: DeleteFcn=PreScanBlockDeleteFcn;
      mask Help: eval('openHelp(733)')
  VISUMatrixSign_HighwayOverhang_1 : Outport  Tag=outport/VisuMatrixSign  SampleTime=1/100
  VISUMatrixSignLights_HighwayOverhang_1 : Outport  Tag=outport/VisuMatrixSignLights  Port=2  SampleTime=1/100
  wires:
  VISUMatrixSign_Mux/1(MatrixSigns) -> VISUMatrixSign_HighwayOverhang_1/1
  VISUMatrixSignLights_Mux/1(VISUMatrixSignLights_HighwayOverhang_1) -> VISUMatrixSignLights_HighwayOverhang_1/1
  Ground_1/1 -> VISUMatrixSignLights_Mux/1(MatrixSign_1)
  Ground_2/1 -> VISUMatrixSignLights_Mux/2(MatrixSign_2)
  Ground_3/1 -> VISUMatrixSignLights_Mux/3(MatrixSign_3)
  Ground_4/1 -> VISUMatrixSignLights_Mux/4(MatrixSign_4)
  Ground_5/1 -> VISUMatrixSign_Mux/1(MatrixSign_1)
  Ground_6/1 -> VISUMatrixSign_Mux/2(MatrixSign_2)
  Ground_7/1 -> VISUMatrixSign_Mux/3(MatrixSign_3)
  Ground_8/1 -> VISUMatrixSign_Mux/4(MatrixSign_4)

== system TSR_Scenario_001_cs/HighwayOverhang_2 ==
  note: Resources
      |
      | 3: InformationSign\MatrixSign_Empty.png: MatrixSign Empty
      | 4: InformationSign\MatrixSign_End.png: MatrixSign End
      | 5: InformationSign\MatrixSign_GreenArrow.png: MatrixSign GreenArrow
      | 6: InformationSign\MatrixSign_RedCross.png: MatrixSign RedCross
      | 7: InformationSign\MatrixSign_Speed_50.png: MatrixSign Speed 50
      | 8: InformationSign\MatrixSign_Speed_70.png: MatrixSign Speed 70
      | 9: InformationSign\MatrixSign_Speed_90.png: MatrixSign Speed 90
      | 10: InformationSign\MatrixSign_Speed_120.png: MatrixSign Speed 120
      | 11: InformationSign\MatrixSign_Speed_130.png: MatrixSign Speed 130
      | 12: InformationSign\information.png: information
      | 13: InformationSign\Empty.jpg: Empty
  Ground_{1..8} (8 alike) : Ground
  VISUMatrixSignLights_Mux : Subsystem  Tag=mux/VisuMatrixSignLights  mask(PreScan User Interface: VisuMatrixSignLights){}
      mask help:
      | The VisuMatrixSignLights block provides a way to switch the lights on the matrix sign board on or off
      |
      | For more information, please click Help.
      mask Help: eval('openHelp(732)')
  VISUMatrixSign_Mux : Subsystem  Tag=mux/MatrixSign_v2  mask(PreScan User Interface: VisuMatrixSign){}
      mask help:
      | The VisuMatrixSign block provides a way to adapt the texture of the plates connected to an overhang, based on Resource IDs of the texture files.
      |
      | For more information, please click Help.
      settings: DeleteFcn=PreScanBlockDeleteFcn;
      mask Help: eval('openHelp(733)')
  VISUMatrixSign_HighwayOverhang_2 : Outport  Tag=outport/VisuMatrixSign  SampleTime=1/100
  VISUMatrixSignLights_HighwayOverhang_2 : Outport  Tag=outport/VisuMatrixSignLights  Port=2  SampleTime=1/100
  wires:
  VISUMatrixSign_Mux/1(MatrixSigns) -> VISUMatrixSign_HighwayOverhang_2/1
  VISUMatrixSignLights_Mux/1(VISUMatrixSignLights_HighwayOverhang_2) -> VISUMatrixSignLights_HighwayOverhang_2/1
  Ground_1/1 -> VISUMatrixSignLights_Mux/1(MatrixSign_5)
  Ground_2/1 -> VISUMatrixSignLights_Mux/2(MatrixSign_6)
  Ground_3/1 -> VISUMatrixSignLights_Mux/3(MatrixSign_7)
  Ground_4/1 -> VISUMatrixSignLights_Mux/4(MatrixSign_8)
  Ground_5/1 -> VISUMatrixSign_Mux/1(MatrixSign_5)
  Ground_6/1 -> VISUMatrixSign_Mux/2(MatrixSign_6)
  Ground_7/1 -> VISUMatrixSign_Mux/3(MatrixSign_7)
  Ground_8/1 -> VISUMatrixSign_Mux/4(MatrixSign_8)

== system TSR_Scenario_001_cs/HighwayOverhang_3 ==
  note: Resources
      |
      | 3: InformationSign\MatrixSign_Empty.png: MatrixSign Empty
      | 4: InformationSign\MatrixSign_End.png: MatrixSign End
      | 5: InformationSign\MatrixSign_GreenArrow.png: MatrixSign GreenArrow
      | 6: InformationSign\MatrixSign_RedCross.png: MatrixSign RedCross
      | 7: InformationSign\MatrixSign_Speed_50.png: MatrixSign Speed 50
      | 8: InformationSign\MatrixSign_Speed_70.png: MatrixSign Speed 70
      | 9: InformationSign\MatrixSign_Speed_90.png: MatrixSign Speed 90
      | 10: InformationSign\MatrixSign_Speed_120.png: MatrixSign Speed 120
      | 11: InformationSign\MatrixSign_Speed_130.png: MatrixSign Speed 130
      | 12: InformationSign\information.png: information
      | 13: InformationSign\Empty.jpg: Empty
  Ground_{1..8} (8 alike) : Ground
  VISUMatrixSignLights_Mux : Subsystem  Tag=mux/VisuMatrixSignLights  mask(PreScan User Interface: VisuMatrixSignLights){}
      mask help:
      | The VisuMatrixSignLights block provides a way to switch the lights on the matrix sign board on or off
      |
      | For more information, please click Help.
      mask Help: eval('openHelp(732)')
  VISUMatrixSign_Mux : Subsystem  Tag=mux/MatrixSign_v2  mask(PreScan User Interface: VisuMatrixSign){}
      mask help:
      | The VisuMatrixSign block provides a way to adapt the texture of the plates connected to an overhang, based on Resource IDs of the texture files.
      |
      | For more information, please click Help.
      settings: DeleteFcn=PreScanBlockDeleteFcn;
      mask Help: eval('openHelp(733)')
  VISUMatrixSign_HighwayOverhang_3 : Outport  Tag=outport/VisuMatrixSign  SampleTime=1/100
  VISUMatrixSignLights_HighwayOverhang_3 : Outport  Tag=outport/VisuMatrixSignLights  Port=2  SampleTime=1/100
  wires:
  VISUMatrixSign_Mux/1(MatrixSigns) -> VISUMatrixSign_HighwayOverhang_3/1
  VISUMatrixSignLights_Mux/1(VISUMatrixSignLights_HighwayOverhang_3) -> VISUMatrixSignLights_HighwayOverhang_3/1
  Ground_1/1 -> VISUMatrixSignLights_Mux/1(MatrixSign_10)
  Ground_2/1 -> VISUMatrixSignLights_Mux/2(MatrixSign_11)
  Ground_3/1 -> VISUMatrixSignLights_Mux/3(MatrixSign_12)
  Ground_4/1 -> VISUMatrixSignLights_Mux/4(MatrixSign_9)
  Ground_5/1 -> VISUMatrixSign_Mux/1(MatrixSign_9)
  Ground_6/1 -> VISUMatrixSign_Mux/2(MatrixSign_10)
  Ground_7/1 -> VISUMatrixSign_Mux/3(MatrixSign_11)
  Ground_8/1 -> VISUMatrixSign_Mux/4(MatrixSign_12)

== system TSR_Scenario_001_cs/HighwayOverhang_4 ==
  note: Resources
      |
      | 3: InformationSign\MatrixSign_Empty.png: MatrixSign Empty
      | 4: InformationSign\MatrixSign_End.png: MatrixSign End
      | 5: InformationSign\MatrixSign_GreenArrow.png: MatrixSign GreenArrow
      | 6: InformationSign\MatrixSign_RedCross.png: MatrixSign RedCross
      | 7: InformationSign\MatrixSign_Speed_50.png: MatrixSign Speed 50
      | 8: InformationSign\MatrixSign_Speed_70.png: MatrixSign Speed 70
      | 9: InformationSign\MatrixSign_Speed_90.png: MatrixSign Speed 90
      | 10: InformationSign\MatrixSign_Speed_120.png: MatrixSign Speed 120
      | 11: InformationSign\MatrixSign_Speed_130.png: MatrixSign Speed 130
      | 12: InformationSign\information.png: information
      | 13: InformationSign\Empty.jpg: Empty
  Ground_{1..8} (8 alike) : Ground
  VISUMatrixSignLights_Mux : Subsystem  Tag=mux/VisuMatrixSignLights  mask(PreScan User Interface: VisuMatrixSignLights){}
      mask help:
      | The VisuMatrixSignLights block provides a way to switch the lights on the matrix sign board on or off
      |
      | For more information, please click Help.
      mask Help: eval('openHelp(732)')
  VISUMatrixSign_Mux : Subsystem  Tag=mux/MatrixSign_v2  mask(PreScan User Interface: VisuMatrixSign){}
      mask help:
      | The VisuMatrixSign block provides a way to adapt the texture of the plates connected to an overhang, based on Resource IDs of the texture files.
      |
      | For more information, please click Help.
      settings: DeleteFcn=PreScanBlockDeleteFcn;
      mask Help: eval('openHelp(733)')
  VISUMatrixSign_HighwayOverhang_4 : Outport  Tag=outport/VisuMatrixSign  SampleTime=1/100
  VISUMatrixSignLights_HighwayOverhang_4 : Outport  Tag=outport/VisuMatrixSignLights  Port=2  SampleTime=1/100
  wires:
  VISUMatrixSign_Mux/1(MatrixSigns) -> VISUMatrixSign_HighwayOverhang_4/1
  VISUMatrixSignLights_Mux/1(VISUMatrixSignLights_HighwayOverhang_4) -> VISUMatrixSignLights_HighwayOverhang_4/1
  Ground_1/1 -> VISUMatrixSignLights_Mux/1(MatrixSign_13)
  Ground_2/1 -> VISUMatrixSignLights_Mux/2(MatrixSign_14)
  Ground_3/1 -> VISUMatrixSignLights_Mux/3(MatrixSign_15)
  Ground_4/1 -> VISUMatrixSignLights_Mux/4(MatrixSign_16)
  Ground_5/1 -> VISUMatrixSign_Mux/1(MatrixSign_13)
  Ground_6/1 -> VISUMatrixSign_Mux/2(MatrixSign_14)
  Ground_7/1 -> VISUMatrixSign_Mux/3(MatrixSign_15)
  Ground_8/1 -> VISUMatrixSign_Mux/4(MatrixSign_16)

== system TSR_Scenario_001_cs/HighwayOverhang_5 ==
  note: Resources
      |
      | 3: InformationSign\MatrixSign_Empty.png: MatrixSign Empty
      | 4: InformationSign\MatrixSign_End.png: MatrixSign End
      | 5: InformationSign\MatrixSign_GreenArrow.png: MatrixSign GreenArrow
      | 6: InformationSign\MatrixSign_RedCross.png: MatrixSign RedCross
      | 7: InformationSign\MatrixSign_Speed_50.png: MatrixSign Speed 50
      | 8: InformationSign\MatrixSign_Speed_70.png: MatrixSign Speed 70
      | 9: InformationSign\MatrixSign_Speed_90.png: MatrixSign Speed 90
      | 10: InformationSign\MatrixSign_Speed_120.png: MatrixSign Speed 120
      | 11: InformationSign\MatrixSign_Speed_130.png: MatrixSign Speed 130
      | 12: InformationSign\information.png: information
      | 13: InformationSign\Empty.jpg: Empty
  Ground_{1..8} (8 alike) : Ground
  VISUMatrixSignLights_Mux : Subsystem  Tag=mux/VisuMatrixSignLights  mask(PreScan User Interface: VisuMatrixSignLights){}
      mask help:
      | The VisuMatrixSignLights block provides a way to switch the lights on the matrix sign board on or off
      |
      | For more information, please click Help.
      mask Help: eval('openHelp(732)')
  VISUMatrixSign_Mux : Subsystem  Tag=mux/MatrixSign_v2  mask(PreScan User Interface: VisuMatrixSign){}
      mask help:
      | The VisuMatrixSign block provides a way to adapt the texture of the plates connected to an overhang, based on Resource IDs of the texture files.
      |
      | For more information, please click Help.
      settings: DeleteFcn=PreScanBlockDeleteFcn;
      mask Help: eval('openHelp(733)')
  VISUMatrixSign_HighwayOverhang_5 : Outport  Tag=outport/VisuMatrixSign  SampleTime=1/100
  VISUMatrixSignLights_HighwayOverhang_5 : Outport  Tag=outport/VisuMatrixSignLights  Port=2  SampleTime=1/100
  wires:
  VISUMatrixSign_Mux/1(MatrixSigns) -> VISUMatrixSign_HighwayOverhang_5/1
  VISUMatrixSignLights_Mux/1(VISUMatrixSignLights_HighwayOverhang_5) -> VISUMatrixSignLights_HighwayOverhang_5/1
  Ground_1/1 -> VISUMatrixSignLights_Mux/1(MatrixSign_17)
  Ground_2/1 -> VISUMatrixSignLights_Mux/2(MatrixSign_18)
  Ground_3/1 -> VISUMatrixSignLights_Mux/3(MatrixSign_19)
  Ground_4/1 -> VISUMatrixSignLights_Mux/4(MatrixSign_20)
  Ground_5/1 -> VISUMatrixSign_Mux/1(MatrixSign_17)
  Ground_6/1 -> VISUMatrixSign_Mux/2(MatrixSign_18)
  Ground_7/1 -> VISUMatrixSign_Mux/3(MatrixSign_19)
  Ground_8/1 -> VISUMatrixSign_Mux/4(MatrixSign_20)
